simulink model "Trajectory_tracking"  (R2016b)
settings: Solver=ode1  StartTime=0.0  StopTime=pre_time + t_fin + post_time  FixedStep=T_sample  MinStep=1e-4  RelTol=1e-3
undefined symbols (not defined in the file): Activator, dx_0, pre_time, t_fin, T_sample, x_0
libraries: simulink x2, qbmove_library x2, QB_pacer_lib x1
settings Model: Creator=Franco  LastModifiedBy=Franco
settings DataIOCC: LimitDataPoints=on  SaveFormat=Array  SignalLoggingSaveFormat=ModelDataLogs
settings OptimizationCC: ExpressionDepthLimit=2147483647  EfficientMapNaN2IntZero=off  LifeSpan=inf
settings DebuggingCC: UnderspecifiedInitializationDetection=Classic  MergeDetectMultiDrivingBlocksExec=none  SolverPrmCheckMsg=warning  FcnCallInpInsideContextMsg=warning  AllowSymbolicDim=off  StateNameClashWarn=warning  SFUnexpectedBacktrackingDiag=warning  SFNoUnconditionalDefaultTransitionDiag=warning  SFExecutionAtInitializationDiag=none
settings HardwareCC: ProdBitPerPointer=32  ProdBitPerSizeT=32  ProdBitPerPtrDiffT=32  ProdLargestAtomicFloat=None  ProdIntDivRoundTo=Undefined  ProdEndianess=Unspecified  ProdWordSize=32  ProdHWDeviceType=32-bit Generic  TargetBitPerPointer=64  TargetBitPerSizeT=64  TargetBitPerPtrDiffT=64  TargetLongLongMode=on  TargetIntDivRoundTo=Zero  TargetEndianess=LittleEndian  TargetWordSize=64  TargetHWDeviceType=MATLAB Host  ProdEqTarget=off
settings ModelReferenceCC: PropagateSignalLabelsOutOfModel=off
settings CodeAppCC: MaxIdLength=128
settings GRTTargetCC: TargetLangStandard=C89/C90 (ANSI)  GeneratePreprocessorConditionals=Disable all  CombineOutputUpdateFcns=off  GRTInterface=on
settings ConfigComp: CovMetricSettings=dw  CovHtmlReporting=on  CovSaveCumulativeToWorkspaceVar=on  CovSaveSingleToWorkspaceVar=on  CovExternalEMLEnable=off  CovSFcnEnable=off
settings ConfigurationSet: Description=SimMechanics 2G

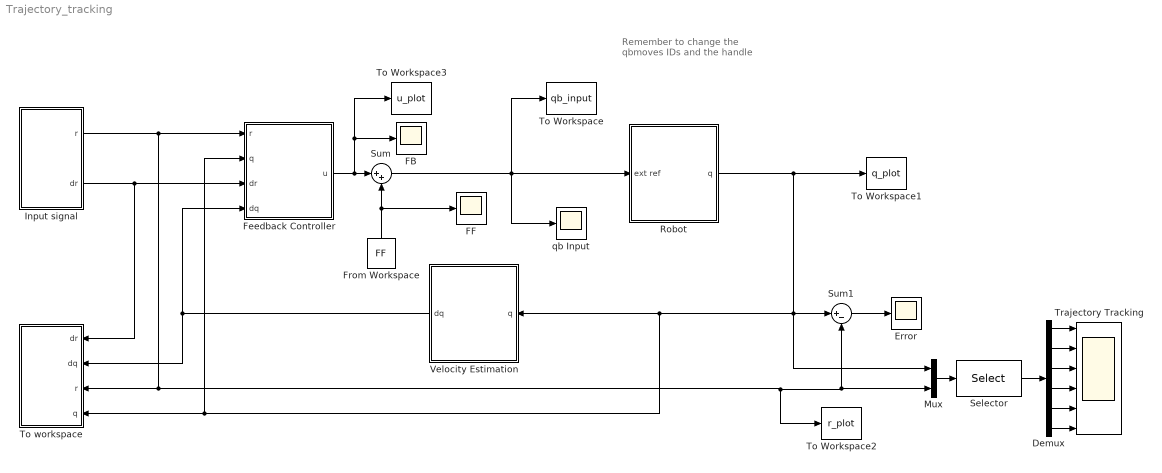
== system Trajectory_tracking ==
  note: Remember to change the qbmoves IDs and the handle
  Demux : Demux  Outputs=[2 2 2 2 2 2]
  Error : Scope
  FB : Scope
  FF : Scope
  Feedback Controller : Subsystem
  From Workspace : FromWorkspace  VariableName=FF  SampleTime=0  OutputAfterFinalValue=Setting to zero
  Input signal : Subsystem
  Mux : Mux  Inputs=2
  Robot : Subsystem
  Selector : Selector  InputPortWidth=12  IndexOptions=Index vector (dialog)  Indices=[1 7 2 8 3 9 4 10 5 11 6 12]  OutputSizes=1
  Sum : Sum  Inputs=|++
  Sum1 : Sum  Inputs=|+-
  To Workspace : ToWorkspace  VariableName=qb_input  SaveFormat=Structure With Time  SampleTime=-1
  To Workspace1 : ToWorkspace  VariableName=q_plot  SaveFormat=Structure With Time  SampleTime=-1
  To Workspace2 : ToWorkspace  VariableName=r_plot  SaveFormat=Structure With Time  SampleTime=-1
  To Workspace3 : ToWorkspace  VariableName=u_plot  SaveFormat=Structure With Time  SampleTime=-1
  To workspace : Subsystem
  Trajectory Tracking : Scope  NumInputPorts=6
  Velocity Estimation : Subsystem
  qb Input : Scope
  wires:
  Feedback Controller/1(u) -> Sum/1, To Workspace3/1, FB/1
  Input signal/2(dr) -> To workspace/1(dr), Feedback Controller/3(dr)
  Input signal/1(r) -> To Workspace2/1, Mux/2, Sum1/2, To workspace/3(r), Feedback Controller/1(r)
  From Workspace/1 -> FF/1, Sum/2
  Sum/1 -> Robot/1("ext ref "), qb Input/1, To Workspace/1
  Velocity Estimation/1(dq) -> Feedback Controller/4(dq), To workspace/2(dq)
  Sum1/1 -> Error/1
  Robot/1(q) -> Mux/1, Sum1/1, To workspace/4(q), Feedback Controller/2(q), Velocity Estimation/1(q), To Workspace1/1
  Mux/1 -> Selector/1
  Selector/1 -> Demux/1
  Demux/1 -> Trajectory Tracking/1
  Demux/2 -> Trajectory Tracking/2
  Demux/3 -> Trajectory Tracking/3
  Demux/4 -> Trajectory Tracking/4
  Demux/5 -> Trajectory Tracking/5
  Demux/6 -> Trajectory Tracking/6

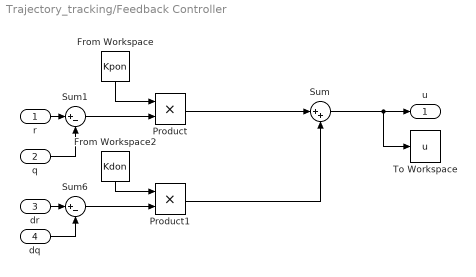
== system Trajectory_tracking/Feedback Controller ==
  r : Inport
  q : Inport  Port=2
  dr : Inport  Port=3
  dq : Inport  Port=4
  From Workspace : FromWorkspace  VariableName=Kpon
  From Workspace2 : FromWorkspace  VariableName=Kdon
  Product : Product
  Product1 : Product
  Sum : Sum  Inputs=|++
  Sum1 : Sum  Inputs=|+-
  Sum6 : Sum  Inputs=|+-
  To Workspace : ToWorkspace  VariableName=u  SaveFormat=Structure With Time  SampleTime=-1
  u : Outport
  wires:
  r/1 -> Sum1/1
  dr/1 -> Sum6/1
  q/1 -> Sum1/2
  dq/1 -> Sum6/2
  Sum/1 -> To Workspace/1, u/1
  Sum6/1 -> Product1/2
  From Workspace/1 -> Product/1
  From Workspace2/1 -> Product1/1
  Sum1/1 -> Product/2
  Product1/1 -> Sum/2
  Product/1 -> Sum/1

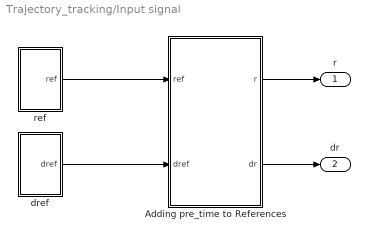
== system Trajectory_tracking/Input signal ==
  Adding pre_time to References : Subsystem
  dref : Subsystem
  ref : Subsystem
  r : Outport
  dr : Outport  Port=2
  wires:
  ref/1(ref) -> Adding pre_time to References/1(ref)
  dref/1(dref) -> Adding pre_time to References/2(dref)
  Adding pre_time to References/1(r) -> r/1
  Adding pre_time to References/2(dr) -> dr/1

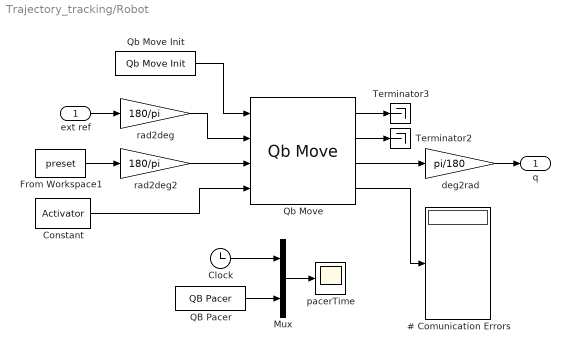
== system Trajectory_tracking/Robot ==
  "ext ref " : Inport
  # Comunication Errors : Display
  Clock : Clock
  Constant : Constant  Value=Activator
  From Workspace1 : FromWorkspace  VariableName=preset  SampleTime=0  OutputAfterFinalValue=Setting to zero
  Mux : Mux  Inputs=2
  QB Pacer : QB_pacer_lib/QB Pacer  simTimePerRealTime=1
  Qb Move : qbmove_library/Qb Move  ID=[1 2 3 4 5 6]  ACTIVE_COMM_DIRECTIONS=Both  CONTROL_MODE=Equilibrium Position and Stiffness Preset  DAISY_CHAINING=off  MAX_ANG=0  SW_LIMIT=inf  OFFSET=0  ACTIVATE=off  WDT=0.0  UNIT=Degrees
  Qb Move Init : qbmove_library/Qb Move Init  NUMBER_OF_COM='COM7'  BAUD_RATE_COM=2000000
  Terminator2 : Terminator
  Terminator3 : Terminator
  deg2rad : Gain  Gain=pi/180
  pacerTime : Scope
  rad2deg : Gain  Gain=180/pi
  rad2deg2 : Gain  Gain=180/pi
  q : Outport
  wires:
  deg2rad/1 -> q/1
  "ext ref "/1 -> rad2deg/1
  QB Pacer/1 -> Mux/2
  Clock/1 -> Mux/1
  Qb Move Init/1 -> Qb Move/1
  Mux/1 -> pacerTime/1
  Qb Move/1 -> Terminator3/1
  Qb Move/2 -> Terminator2/1
  Qb Move/3 -> deg2rad/1
  rad2deg/1 -> Qb Move/2
  Qb Move/4 -> # Comunication Errors/1
  rad2deg2/1 -> Qb Move/3
  Constant/1 -> Qb Move/4
  From Workspace1/1 -> rad2deg2/1

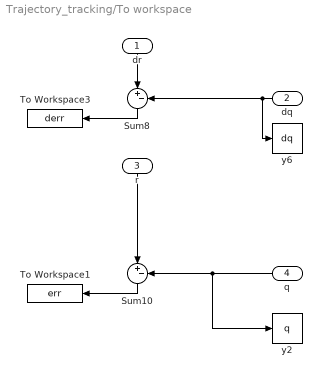
== system Trajectory_tracking/To workspace ==
  dr : Inport
  dq : Inport  Port=2
  r : Inport  Port=3
  q : Inport  Port=4
  Sum10 : Sum  Inputs=|+-
  Sum8 : Sum  Inputs=|+-
  To Workspace1 : ToWorkspace  VariableName=err  SaveFormat=Structure With Time  SampleTime=-1
  To Workspace3 : ToWorkspace  VariableName=derr  SaveFormat=Structure With Time  SampleTime=-1
  y2 : ToWorkspace  VariableName=q  SaveFormat=Structure With Time  SampleTime=-1
  y6 : ToWorkspace  VariableName=dq  SaveFormat=Structure With Time  SampleTime=-1
  wires:
  dq/1 -> y6/1, Sum8/2
  q/1 -> Sum10/2, y2/1
  Sum8/1 -> To Workspace3/1
  dr/1 -> Sum8/1
  r/1 -> Sum10/1
  Sum10/1 -> To Workspace1/1

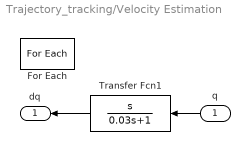
== system Trajectory_tracking/Velocity Estimation ==
  q : Inport  Partition=on  PartitionDimension=1  PartitionWidth=1
  For Each : ForEach  DisableCoverage=on  IndexMode=One-based
  Transfer Fcn1 : TransferFcn  Numerator=[1 0]  Denominator=[0.03 1]
  dq : Outport  ConcatenationDimension=1
  wires:
  q/1 -> Transfer Fcn1/1
  Transfer Fcn1/1 -> dq/1

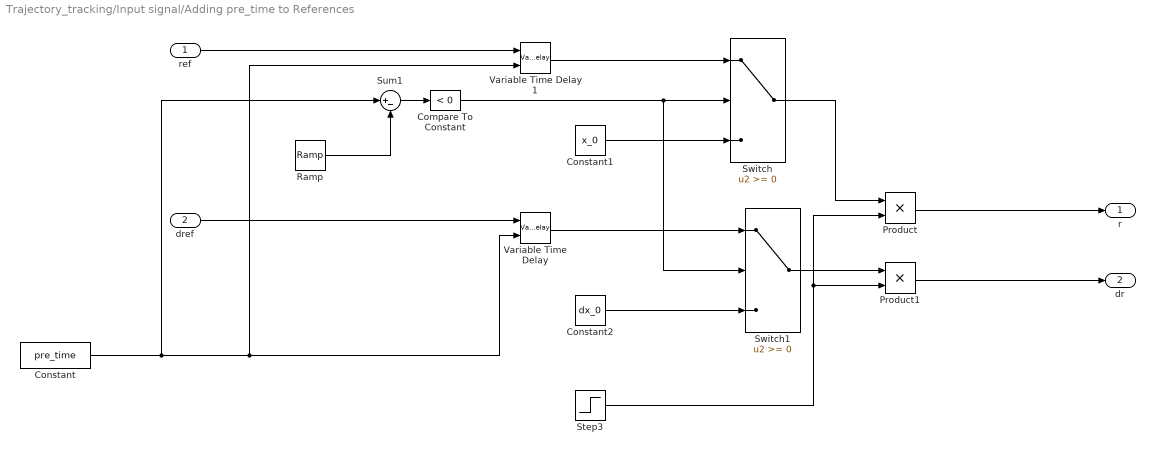
== system Trajectory_tracking/Input signal/Adding pre_time to References ==
  ref : Inport
  dref : Inport  Port=2
  Compare To Constant : simulink/Logic and Bit Operations/Compare To Constant  relop=<  const=0  OutDataTypeStr=boolean
  Constant : Constant  Value=pre_time
  Constant1 : Constant  Value=x_0
  Constant2 : Constant  Value=dx_0
  Product : Product
  Product1 : Product
  Ramp : simulink/Sources/Ramp  slope=1  start=0  X0=0
  Step3 : Step  Time=t_fin + pre_time + T_sample  Before=1  After=0  SampleTime=0
  Sum1 : Sum  Inputs=|+-
  Switch : Switch
  Switch1 : Switch
  Variable Time Delay : VariableTransportDelay  MaximumDelay=pre_time  MaximumPoints=4096
  Variable Time Delay 1 : VariableTransportDelay  MaximumDelay=pre_time  MaximumPoints=4096
  r : Outport
  dr : Outport  Port=2
  wires:
  Constant/1 -> Variable Time Delay/2, Variable Time Delay 1/2, Sum1/1
  Sum1/1 -> Compare To Constant/1
  dref/1 -> Variable Time Delay/1
  Step3/1 -> Product/2, Product1/2
  Variable Time Delay/1 -> Switch1/1
  Ramp/1 -> Sum1/2
  Compare To Constant/1 -> Switch1/2, Switch/2
  Variable Time Delay 1/1 -> Switch/1
  ref/1 -> Variable Time Delay 1/1
  Product/1 -> r/1
  Product1/1 -> dr/1
  Switch1/1 -> Product1/1
  Constant2/1 -> Switch1/3
  Switch/1 -> Product/1
  Constant1/1 -> Switch/3

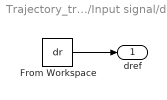
== system Trajectory_tracking/Input signal/dref ==
  From Workspace : FromWorkspace  VariableName=dr  SampleTime=0  OutputAfterFinalValue=Setting to zero
  dref : Outport
  wires:
  From Workspace/1 -> dref/1

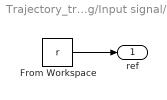
== system Trajectory_tracking/Input signal/ref ==
  From Workspace : FromWorkspace  VariableName=r  SampleTime=0  OutputAfterFinalValue=Setting to zero
  ref : Outport
  wires:
  From Workspace/1 -> ref/1
